simulink library "MSMLib"  (R2018b)
settings: Solver=VariableStepAuto  StartTime=0.0  StopTime=10.0  RelTol=1e-3
undefined symbols (not defined in the file or in its folder): MdTp1, ModeAdjustTp1, PosCallSts1
settings Model: Creator=s69u2m  LastModifiedBy=su3dcu
settings DataIOCC: ReturnWorkspaceOutputs=on

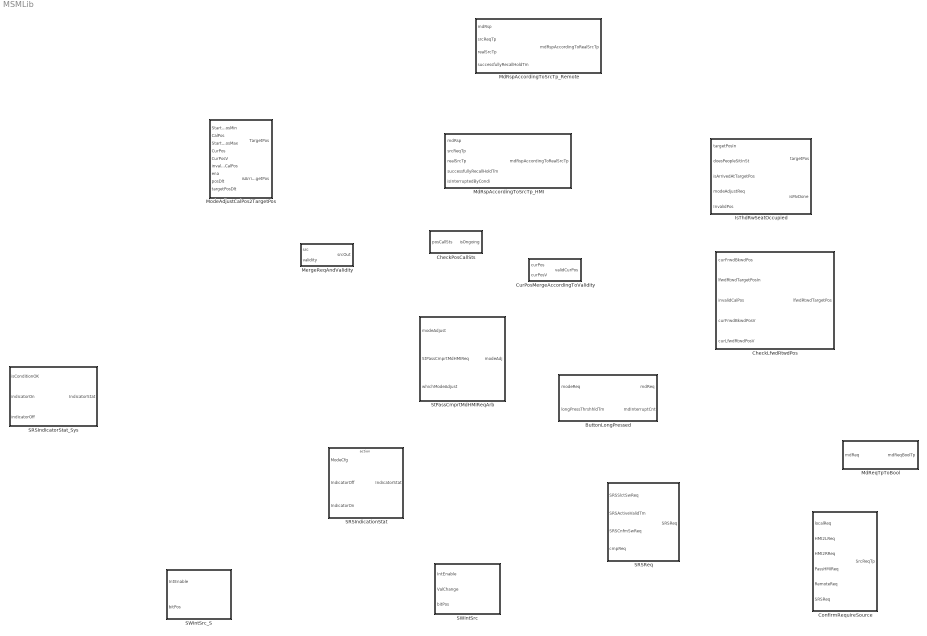
== system MSMLib ==
  ButtonLongPressed : Subsystem
  CheckLfwdRtwdPos : Subsystem
  CheckPosCallSts : Subsystem
  ConfirmRequireSource : Subsystem
  CurPosMergeAccordingToValidity : Subsystem
  IsThdRwSeatOccupied : Subsystem
  MdReqTpToBool : Subsystem
  MdRspAccordingToSrcTp_HMI : Subsystem
  MdRspAccordingToSrcTp_Remote : Subsystem
  MergeReqAndValidity : Subsystem
  ModeAdjustCalPos2TargetPos : Subsystem
  "SRSIndicationStat " : Subsystem  TreatAsAtomicUnit=on
  SRSIndicatorStat_Sys : Subsystem
  SRSReq : Subsystem
  SWIntSrc : Subsystem
  SWIntSrc_S : Subsystem
  StPassCmprtMdHMIReqArb : Subsystem

== system MSMLib/ButtonLongPressed ==
  modeReq : Inport
  longPressThrshhldTm : Inport  Port=2
  Chart1 : Stateflow chart  TreatAsAtomicUnit=on
  mdReq : Outport
  mdInterruptCnt : Outport  Port=2
  wires:
  longPressThrshhldTm/1 -> Chart1/2(iLongPressThrshhldTm)
  Chart1/2(oMdInterruptCnt) -> mdInterruptCnt/1
  Chart1/1(oMdReq) -> mdReq/1
  modeReq/1 -> Chart1/1(iSrc)

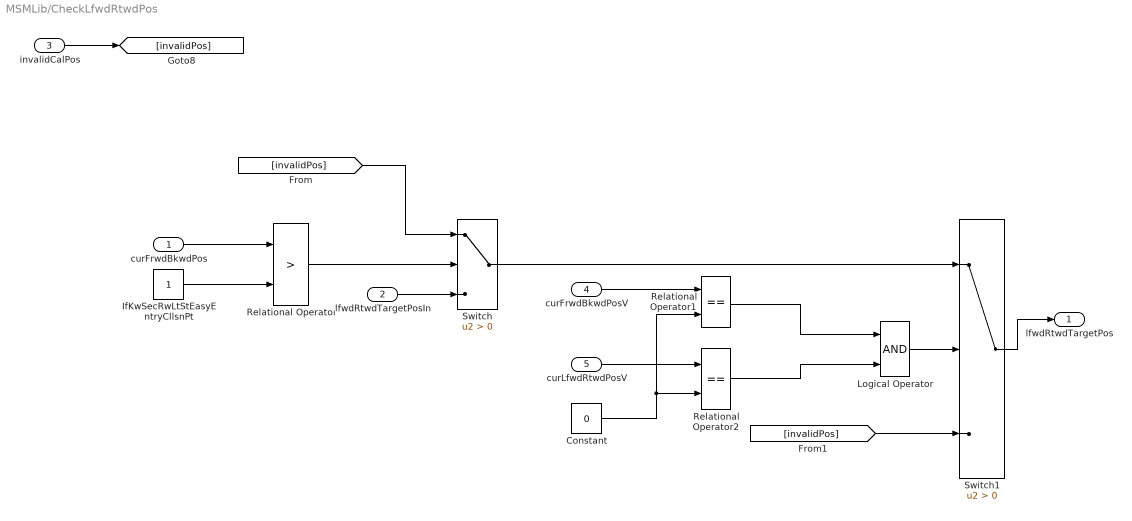
== system MSMLib/CheckLfwdRtwdPos ==
  curFrwdBkwdPos : Inport
  lfwdRtwdTargetPosIn : Inport  Port=2
  invalidCalPos : Inport  Port=3
  curFrwdBkwdPosV : Inport  Port=4
  curLfwdRtwdPosV : Inport  Port=5
  Constant : Constant  Value=0  OutDataTypeStr=uint8
  IfKwSecRwLtStEasyEntryCllsnPt : Constant  OutDataTypeStr=uint16
  Logical Operator : Logic  AllPortsSameDT=off  OutDataTypeStr=boolean
  Relational Operator : RelationalOperator  Operator=>  OutDataTypeStr=boolean  RndMeth=Simplest
  Relational Operator1 : RelationalOperator  Operator===  OutDataTypeStr=boolean  RndMeth=Simplest
  Relational Operator2 : RelationalOperator  Operator===  OutDataTypeStr=boolean  RndMeth=Simplest
  Switch : Switch  Criteria=u2 > Threshold
  Switch1 : Switch  Criteria=u2 > Threshold
  lfwdRtwdTargetPos : Outport  VectorParamsAs1DForOutWhenUnconnected=on
  wires:
  Logical Operator/1 -> Switch1/2
  Relational Operator2/1 -> Logical Operator/2
  curLfwdRtwdPosV/1 -> Relational Operator2/1
  [invalidPos] -> Switch1/3
  Relational Operator1/1 -> Logical Operator/1
  Switch1/1 -> lfwdRtwdTargetPos/1
  Switch/1 -> Switch1/1
  [invalidPos] -> Switch/1
  lfwdRtwdTargetPosIn/1 -> Switch/3
  Relational Operator/1 -> Switch/2
  invalidCalPos/1 -> [invalidPos]
  IfKwSecRwLtStEasyEntryCllsnPt/1 -> Relational Operator/2
  curFrwdBkwdPos/1 -> Relational Operator/1
  curFrwdBkwdPosV/1 -> Relational Operator1/1
  Constant/1 -> Relational Operator1/2, Relational Operator2/2

== system MSMLib/CheckPosCallSts ==
  posCallSts : Inport
  Constant : Constant  Value=PosCallSts1.PosCallSts_Ongoing  OutDataTypeStr=Enum:PosCallSts1
  Relational Operator : RelationalOperator  Operator===  OutDataTypeStr=boolean  RndMeth=Simplest
  isOngoing : Outport  VectorParamsAs1DForOutWhenUnconnected=on
  wires:
  Constant/1 -> Relational Operator/2
  posCallSts/1 -> Relational Operator/1
  Relational Operator/1 -> isOngoing/1

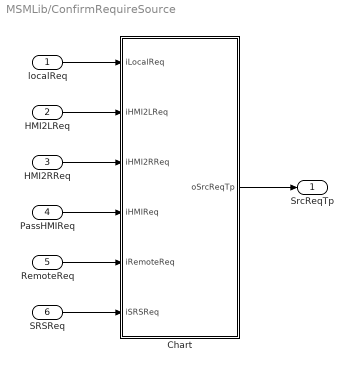
== system MSMLib/ConfirmRequireSource ==
  localReq : Inport
  HMI2LReq : Inport  Port=2
  HMI2RReq : Inport  Port=3
  PassHMIReq : Inport  Port=4
  RemoteReq : Inport  Port=5
  SRSReq : Inport  Port=6
  Chart : Stateflow chart  TreatAsAtomicUnit=on
  SrcReqTp : Outport
  wires:
  HMI2LReq/1 -> Chart/2(iHMI2LReq)
  localReq/1 -> Chart/1(iLocalReq)
  Chart/1(oSrcReqTp) -> SrcReqTp/1
  PassHMIReq/1 -> Chart/4(iHMIReq)
  HMI2RReq/1 -> Chart/3(iHMI2RReq)
  RemoteReq/1 -> Chart/5(iRemoteReq)
  SRSReq/1 -> Chart/6(iSRSReq)

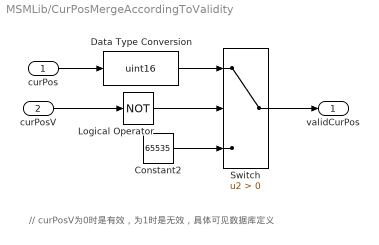
== system MSMLib/CurPosMergeAccordingToValidity ==
  note: // curPosV为0时是有效，为1时是无效，具体可见数据库定义
  curPos : Inport
  curPosV : Inport  Port=2
  Constant2 : Constant  Value=65535  OutDataTypeStr=uint16
  Data Type Conversion : DataTypeConversion  OutDataTypeStr=uint16
  Logical Operator : Logic  Operator=NOT  AllPortsSameDT=off  OutDataTypeStr=boolean
  Switch : Switch  Criteria=u2 > Threshold
  validCurPos : Outport  VectorParamsAs1DForOutWhenUnconnected=on
  wires:
  Constant2/1 -> Switch/3
  Logical Operator/1 -> Switch/2
  Data Type Conversion/1 -> Switch/1
  curPos/1 -> Data Type Conversion/1
  curPosV/1 -> Logical Operator/1
  Switch/1 -> validCurPos/1

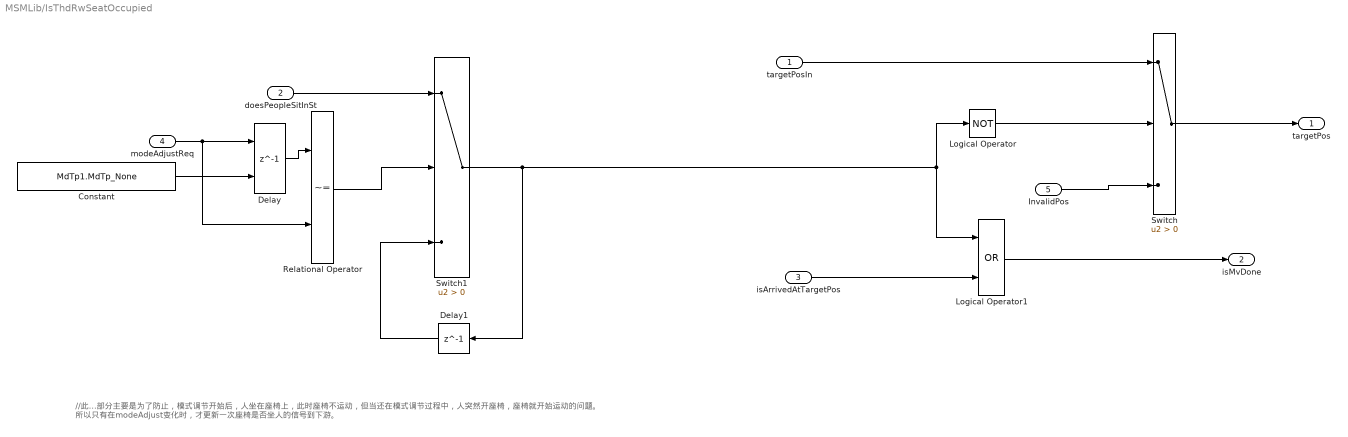
== system MSMLib/IsThdRwSeatOccupied ==
  note: //此部分主要是为了防止，模式调节开始后，人坐在座椅上，此时座椅不运动，但当还在模式调节过程中，人突然开座椅，座椅就开始运动的问题。
      | 所以只有在modeAdjust变化时，才更新一次座椅是否坐人的信号到下游。
  targetPosIn : Inport
  doesPeopleSitInSt : Inport  Port=2
  isArrivedAtTargetPos : Inport  Port=3
  modeAdjustReq : Inport  Port=4
  InvalidPos : Inport  Port=5
  Constant : Constant  Value=MdTp1.MdTp_None  OutDataTypeStr=Enum:MdTp1
  Delay : Delay  DelayLength=1  InitialConditionSource=Input port
      settings: InputPortMap=u0,p4
  Delay1 : Delay  DelayLength=1
  Logical Operator : Logic  Operator=NOT  AllPortsSameDT=off  OutDataTypeStr=boolean
  Logical Operator1 : Logic  Operator=OR  AllPortsSameDT=off  OutDataTypeStr=boolean
  Relational Operator : RelationalOperator  Operator=~=  OutDataTypeStr=boolean  RndMeth=Simplest
  Switch : Switch  Criteria=u2 > Threshold
  Switch1 : Switch  Criteria=u2 > Threshold
  targetPos : Outport  VectorParamsAs1DForOutWhenUnconnected=on
  isMvDone : Outport  Port=2  VectorParamsAs1DForOutWhenUnconnected=on
  wires:
  Switch/1 -> targetPos/1
  Logical Operator1/1 -> isMvDone/1
  isArrivedAtTargetPos/1 -> Logical Operator1/2
  InvalidPos/1 -> Switch/3
  Logical Operator/1 -> Switch/2
  targetPosIn/1 -> Switch/1
  modeAdjustReq/1 -> Relational Operator/2, Delay/1
  Delay/1 -> Relational Operator/1
  Relational Operator/1 -> Switch1/2
  doesPeopleSitInSt/1 -> Switch1/1
  Switch1/1 -> Logical Operator/1, Logical Operator1/1, Delay1/1
  Delay1/1 -> Switch1/3
  Constant/1 -> Delay/2

== system MSMLib/MdReqTpToBool ==
  mdReq : Inport
  Chart : Stateflow chart  TreatAsAtomicUnit=on
  mdReqBoolTp : Outport
  wires:
  Chart/1(oMdReqBool) -> mdReqBoolTp/1
  mdReq/1 -> Chart/1(iMdReq)

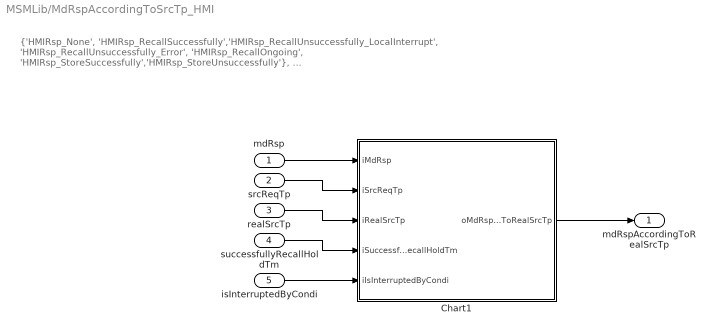
== system MSMLib/MdRspAccordingToSrcTp_HMI ==
  note: {'HMIRsp_None', 'HMIRsp_RecallSuccessfully','HMIRsp_RecallUnsuccessfully_LocalInterrupt', 'HMIRsp_RecallUnsuccessfully_Error', 'HMIRsp_RecallOngoing', 'HMIRsp_StoreSuccessfully','HMIRsp_StoreUnsuccessfully'}, ...
  mdRsp : Inport
  srcReqTp : Inport  Port=2
  realSrcTp : Inport  Port=3
  successfullyRecallHoldTm : Inport  Port=4
  isInterruptedByCondi : Inport  Port=5
  Chart1 : Stateflow chart  TreatAsAtomicUnit=on
  mdRspAccordingToRealSrcTp : Outport
  wires:
  mdRsp/1 -> Chart1/1(iMdRsp)
  srcReqTp/1 -> Chart1/2(iSrcReqTp)
  realSrcTp/1 -> Chart1/3(iRealSrcTp)
  successfullyRecallHoldTm/1 -> Chart1/4(iSuccessfulRecallHoldTm)
  Chart1/1(oMdRspAccordingToRealSrcTp) -> mdRspAccordingToRealSrcTp/1
  isInterruptedByCondi/1 -> Chart1/5(iIsInterruptedByCondi)

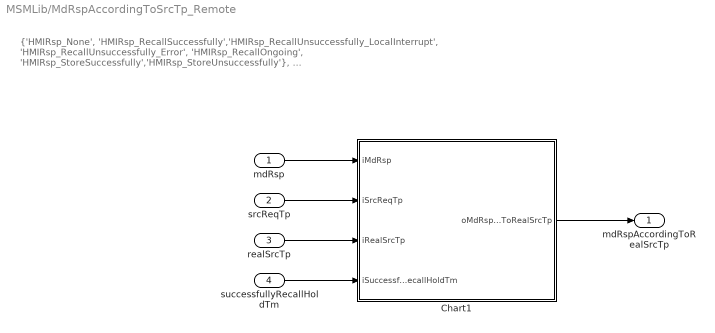
== system MSMLib/MdRspAccordingToSrcTp_Remote ==
  note: {'HMIRsp_None', 'HMIRsp_RecallSuccessfully','HMIRsp_RecallUnsuccessfully_LocalInterrupt', 'HMIRsp_RecallUnsuccessfully_Error', 'HMIRsp_RecallOngoing', 'HMIRsp_StoreSuccessfully','HMIRsp_StoreUnsuccessfully'}, ...
  mdRsp : Inport
  srcReqTp : Inport  Port=2
  realSrcTp : Inport  Port=3
  successfullyRecallHoldTm : Inport  Port=4
  Chart1 : Stateflow chart  TreatAsAtomicUnit=on
  mdRspAccordingToRealSrcTp : Outport
  wires:
  Chart1/1(oMdRspAccordingToRealSrcTp) -> mdRspAccordingToRealSrcTp/1
  successfullyRecallHoldTm/1 -> Chart1/4(iSuccessfulRecallHoldTm)
  realSrcTp/1 -> Chart1/3(iRealSrcTp)
  srcReqTp/1 -> Chart1/2(iSrcReqTp)
  mdRsp/1 -> Chart1/1(iMdRsp)

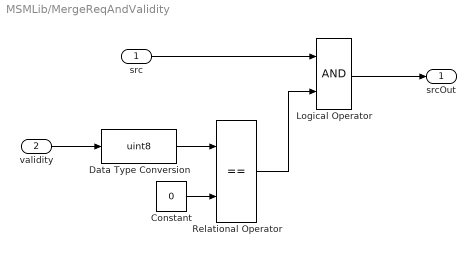
== system MSMLib/MergeReqAndValidity ==
  src : Inport
  validity : Inport  Port=2
  Constant : Constant  Value=0  OutDataTypeStr=uint8
  Data Type Conversion : DataTypeConversion  OutDataTypeStr=uint8
  Logical Operator : Logic  AllPortsSameDT=off  OutDataTypeStr=boolean
  Relational Operator : RelationalOperator  Operator===  OutDataTypeStr=boolean  RndMeth=Simplest
  srcOut : Outport  VectorParamsAs1DForOutWhenUnconnected=on
  wires:
  Relational Operator/1 -> Logical Operator/2
  Logical Operator/1 -> srcOut/1
  validity/1 -> Data Type Conversion/1
  Constant/1 -> Relational Operator/2
  src/1 -> Logical Operator/1
  Data Type Conversion/1 -> Relational Operator/1

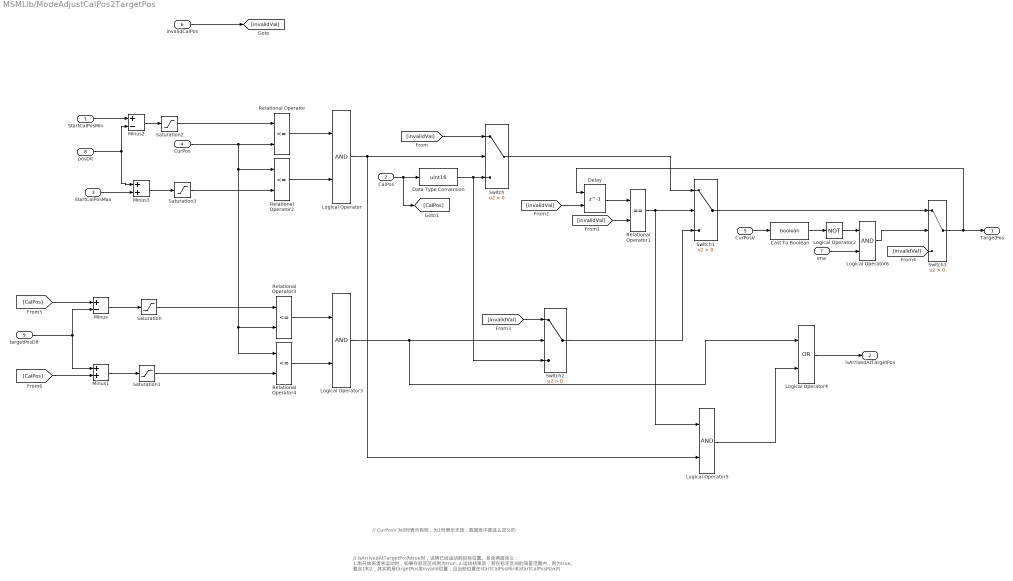
== system MSMLib/ModeAdjustCalPos2TargetPos ==
  note: // isArrivedAtTargetPos为true时，说明已经运动到目标位置。包含两层含义：
      | 1.刚开始来请求运动时，如果在标定区间则为true;
      | 2.运动结束后，若在标定区间的误差范围内，则为true。
      | 整合1和2，其实就是targetPos发invalid位置，且当前位置在startCalPosMin和startCalPosMax内
  note: // CurPosV 为0时表示有效，为1时表示无效，数据库中是这么定义的
  StartCalPosMin : Inport
  CalPos : Inport  Port=2
  StartCalPosMax : Inport  Port=3
  CurPos : Inport  Port=4
  CurPosV : Inport  Port=5
  invalidCalPos : Inport  Port=6
  ena : Inport  Port=7
  posDlt : Inport  Port=8
  targetPosDlt : Inport  Port=9
  Cast To Boolean : DataTypeConversion  OutDataTypeStr=boolean
  Data Type Conversion : DataTypeConversion  OutDataTypeStr=uint16
  Delay : Delay  DelayLength=1  InitialConditionSource=Input port
      settings: InputPortMap=u0,p4
  Logical Operator{,3,5..6} (4 alike) : Logic  AllPortsSameDT=off  OutDataTypeStr=boolean
  Logical Operator2 : Logic  Operator=NOT  AllPortsSameDT=off  OutDataTypeStr=boolean
  Logical Operator4 : Logic  Operator=OR  AllPortsSameDT=off  OutDataTypeStr=boolean
  Minus : Sum  Inputs=+-  OutDataTypeStr=int16
  Minus1 : Sum  OutDataTypeStr=int16
  Minus2 : Sum  Inputs=+-  OutDataTypeStr=int16
  Minus3 : Sum  OutDataTypeStr=uint16
  Relational Operator{,2..4} (4 alike) : RelationalOperator  Operator=<=  OutDataTypeStr=boolean  RndMeth=Simplest
  Relational Operator1 : RelationalOperator  Operator===  OutDataTypeStr=boolean  RndMeth=Simplest
  Saturation : Saturate  UpperLimit=4000  LowerLimit=0  OutDataTypeStr=uint16
  Saturation1 : Saturate  UpperLimit=4000  LowerLimit=0  OutDataTypeStr=uint16
  Saturation2 : Saturate  UpperLimit=4095  LowerLimit=0  OutDataTypeStr=uint16
  Saturation3 : Saturate  UpperLimit=4095  LowerLimit=0  OutDataTypeStr=uint16
  Switch{,1..3} (4 alike) : Switch  Criteria=u2 > Threshold
  TargetPos : Outport  VectorParamsAs1DForOutWhenUnconnected=on
  isArrivedAtTargetPos : Outport  Port=2  VectorParamsAs1DForOutWhenUnconnected=on
  wires:
  StartCalPosMin/1 -> Minus2/1
  Relational Operator/1 -> Logical Operator/1
  StartCalPosMax/1 -> Minus3/2
  Relational Operator2/1 -> Logical Operator/2
  [invalidVal] -> Switch/1
  Logical Operator/1 -> Logical Operator5/2, Switch/2
  Switch/1 -> Switch1/1
  CurPosV/1 -> Cast To Boolean/1
  Cast To Boolean/1 -> Logical Operator2/1
  CalPos/1 -> [CalPos], Data Type Conversion/1
  Delay/1 -> Relational Operator1/1
  Relational Operator1/1 -> Logical Operator5/1, Switch1/2
  Relational Operator3/1 -> Logical Operator3/1
  Relational Operator4/1 -> Logical Operator3/2
  Saturation1/1 -> Relational Operator4/2
  CurPos/1 -> Relational Operator2/1, Relational Operator3/2, Relational Operator4/1, Relational Operator/2
  Saturation/1 -> Relational Operator3/1
  Logical Operator3/1 -> Logical Operator4/1, Switch2/2
  Switch2/1 -> Switch1/3
  Switch1/1 -> Switch3/1
  invalidCalPos/1 -> [invalidVal]
  [invalidVal] -> Relational Operator1/2
  [invalidVal] -> Delay/2
  [invalidVal] -> Switch2/1
  Logical Operator2/1 -> Logical Operator6/1
  [invalidVal] -> Switch3/3
  Data Type Conversion/1 -> Switch/3, Switch2/3
  [CalPos] -> Minus/1
  [CalPos] -> Minus1/2
  Minus/1 -> Saturation/1
  Minus1/1 -> Saturation1/1
  Logical Operator4/1 -> isArrivedAtTargetPos/1
  Logical Operator5/1 -> Logical Operator4/2
  ena/1 -> Logical Operator6/2
  Switch3/1 -> Delay/1, TargetPos/1
  Logical Operator6/1 -> Switch3/2
  targetPosDlt/1 -> Minus1/1, Minus/2
  posDlt/1 -> Minus2/2, Minus3/1
  Minus2/1 -> Saturation2/1
  Saturation2/1 -> Relational Operator/1
  Minus3/1 -> Saturation3/1
  Saturation3/1 -> Relational Operator2/2

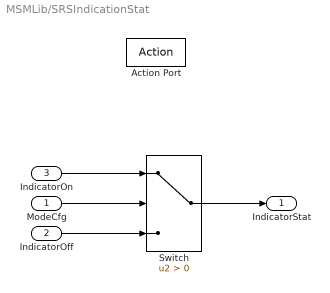
== system MSMLib/SRSIndicationStat  ==
  "ModeCfg " : Inport
  IndicatorOff : Inport  Port=2
  IndicatorOn : Inport  Port=3
  Action Port : ActionPort
  Switch : Switch  Criteria=u2 > Threshold
  "IndicatorStat " : Outport
  wires:
  IndicatorOn/1 -> Switch/1
  "ModeCfg "/1 -> Switch/2
  IndicatorOff/1 -> Switch/3
  Switch/1 -> "IndicatorStat "/1

== system MSMLib/SRSIndicatorStat_Sys ==
  isConditionOK : Inport
  indicatorOn : Inport  Port=2
  indicatorOff : Inport  Port=3
  IndicatorStat_Chart : Stateflow chart  TreatAsAtomicUnit=on
  IndicatorStat : Outport
  wires:
  isConditionOK/1 -> IndicatorStat_Chart/1(isConditionOK)
  indicatorOn/1 -> IndicatorStat_Chart/2(iIndicatorOn)
  indicatorOff/1 -> IndicatorStat_Chart/3(iIndicatorOff)
  IndicatorStat_Chart/1(oIndicatorStat) -> IndicatorStat/1

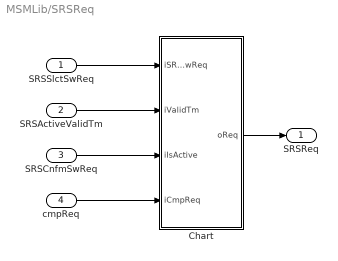
== system MSMLib/SRSReq ==
  SRSSlctSwReq : Inport
  SRSActiveValidTm : Inport  Port=2
  SRSCnfmSwReq : Inport  Port=3
  cmpReq : Inport  Port=4
  Chart : Stateflow chart  TreatAsAtomicUnit=on
  SRSReq : Outport
  wires:
  SRSSlctSwReq/1 -> Chart/1(iSRSSlcSwReq)
  SRSActiveValidTm/1 -> Chart/2(iValidTm)
  SRSCnfmSwReq/1 -> Chart/3(iIsActive)
  cmpReq/1 -> Chart/4(iCmpReq)
  Chart/1(oReq) -> SRSReq/1

== system MSMLib/SWIntSrc ==
  IntEnable : Inport
  "ValChange " : Inport  Port=2
  bitPos : Inport  Port=3
  Chart : Stateflow chart  TreatAsAtomicUnit=on
  wires:
  "ValChange "/1 -> Chart/2(iValChange)
  IntEnable/1 -> Chart/1(iIntEnable)
  bitPos/1 -> Chart/3(ibit)

== system MSMLib/SWIntSrc_S ==
  IntEnable : Inport
  bitPos : Inport  Port=2
  Chart : Stateflow chart  TreatAsAtomicUnit=on
  wires:
  bitPos/1 -> Chart/2(ibit)
  IntEnable/1 -> Chart/1(iIntEnable)

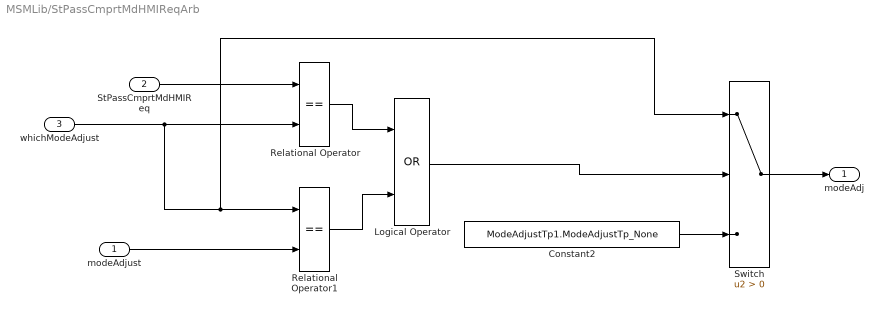
== system MSMLib/StPassCmprtMdHMIReqArb ==
  modeAdjust : Inport
  StPassCmprtMdHMIReq : Inport  Port=2
  whichModeAdjust : Inport  Port=3
  Constant2 : Constant  Value=ModeAdjustTp1.ModeAdjustTp_None  OutDataTypeStr=Enum:ModeAdjustTp1
  Logical Operator : Logic  Operator=OR  AllPortsSameDT=off  OutDataTypeStr=boolean
  Relational Operator : RelationalOperator  Operator===  OutDataTypeStr=boolean  RndMeth=Simplest
  Relational Operator1 : RelationalOperator  Operator===  OutDataTypeStr=boolean  RndMeth=Simplest
  Switch : Switch  Criteria=u2 > Threshold
  modeAdj : Outport  VectorParamsAs1DForOutWhenUnconnected=on
  wires:
  Relational Operator/1 -> Logical Operator/1
  StPassCmprtMdHMIReq/1 -> Relational Operator/1
  Switch/1 -> modeAdj/1
  whichModeAdjust/1 -> Switch/1, Relational Operator1/1, Relational Operator/2
  modeAdjust/1 -> Relational Operator1/2
  Relational Operator1/1 -> Logical Operator/2
  Logical Operator/1 -> Switch/2
  Constant2/1 -> Switch/3

== system MSMLib/SWIntSrc/Chart/MdSWIntSrc_Get ==
  f : TriggerPort  TriggerType=function-call  VariantControl=(inherit)
      settings: CopyFcn=Stateflow.SLINSF.SimulinkMan.removeBlockPreDeleteFcn  PreDeleteFcn=Stateflow.SLINSF.SimulinkMan.unsafePredeleteFcn
  Data Store Read : DataStoreRead  DataStoreName=MdSWIntSrc_Val
  data : Outport  OutDataTypeStr=uint16  PortDimensions=1  SampleTime=0.01
  wires:
  Data Store Read/1 -> data/1

== system MSMLib/SWIntSrc/Chart/MdSWIntSrc_Set ==
  data : Inport  OutDataTypeStr=uint16  PortDimensions=1  SampleTime=0.01
  f : TriggerPort  TriggerType=function-call  VariantControl=(inherit)
      settings: CopyFcn=Stateflow.SLINSF.SimulinkMan.removeBlockPreDeleteFcn  PreDeleteFcn=Stateflow.SLINSF.SimulinkMan.unsafePredeleteFcn
  Data Store Write : DataStoreWrite  DataStoreName=MdSWIntSrc_Val
  wires:
  data/1 -> Data Store Write/1

== system MSMLib/SWIntSrc_S/Chart/MdSWIntSrc_Get ==
  f : TriggerPort  TriggerType=function-call  VariantControl=(inherit)
      settings: CopyFcn=Stateflow.SLINSF.SimulinkMan.removeBlockPreDeleteFcn  PreDeleteFcn=Stateflow.SLINSF.SimulinkMan.unsafePredeleteFcn
  Data Store Read : DataStoreRead  DataStoreName=MdSWIntSrc_Val
  data : Outport  OutDataTypeStr=uint16  PortDimensions=1  SampleTime=0.01
  wires:
  Data Store Read/1 -> data/1

== system MSMLib/SWIntSrc_S/Chart/MdSWIntSrc_Set ==
  data : Inport  OutDataTypeStr=uint16  PortDimensions=1  SampleTime=0.01
  f : TriggerPort  TriggerType=function-call  VariantControl=(inherit)
      settings: CopyFcn=Stateflow.SLINSF.SimulinkMan.removeBlockPreDeleteFcn  PreDeleteFcn=Stateflow.SLINSF.SimulinkMan.unsafePredeleteFcn
  Data Store Write : DataStoreWrite  DataStoreName=MdSWIntSrc_Val
  wires:
  data/1 -> Data Store Write/1

== stateflow chart MSMLib/MdRspAccordingToSrcTp_HMI/Chart1 ==
  state RealSrcTp
    state None
      en:
      oMdRspAccordingToRealSrcTp = HMIRsp1.HMIRsp_None;
    state Ongoing
      en:
      oMdRspAccordingToRealSrcTp = HMIRsp1.HMIRsp_RecallOngoing;
    state successful
      en:
      oMdRspAccordingToRealSrcTp = HMIRsp1.HMIRsp_RecallSuccessfully;
    state Unsuccessful
      state Unsuccess
      (default) -> (junction 41)
      (junction 41) -> Unsuccess [order 1] : [iIsInterruptedByCondi]
          | {oMdRspAccordingToRealSrcTp = HMIRsp1.HMIRsp_RecallUnsuccessfully_Error;}
      (junction 41) -> (junction 43) [order 2]
      (junction 43) -> Unsuccess : {oMdRspAccordingToRealSrcTp = HMIRsp1.HMIRsp_RecallUnsuccessfully_LocalInterrupt;}
    (default) -> (junction 20)
    (junction 20) -> None [order 2]
    (junction 20) -> Ongoing [order 1] : [iMdRsp == MdRsp1.MdRsp_RecallOngoing]
    None -> Ongoing : [iMdRsp == MdRsp1.MdRsp_RecallOngoing]
    Ongoing -> Unsuccessful [order 1] : [iMdRsp == MdRsp1.MdRsp_RecallUnsuccessfully]
    Ongoing -> successful [order 2] : [iMdRsp == MdRsp1.MdRsp_RecallSuccessfully]
    Ongoing -> Unsuccess [order 3] : [iSrcReqTp!=iRealSrcTp]
        | {oMdRspAccordingToRealSrcTp = HMIRsp1.HMIRsp_RecallUnsuccessfully_LocalInterrupt}
    successful -> (junction 35) : [after(iSuccessfulRecallHoldTm,tick)]
    Unsuccessful -> (junction 35) : [after(iSuccessfulRecallHoldTm,tick)]
  state Idle
    en:
    oMdRspAccordingToRealSrcTp = MdRsp1.MdRsp_None;
  (default) -> Idle
  Idle -> RealSrcTp : [iSrcReqTp== iRealSrcTp]
  (junction 35) -> Idle
  data: iMdRsp input Enum: MdRsp1; iSrcReqTp input Enum: SrcReqTp1; oMdRspAccordingToRealSrcTp output Enum: HMIRsp1; iRealSrcTp input Enum: SrcReqTp1; iSuccessfulRecallHoldTm input uint8; iIsInterruptedByCondi input boolean

== stateflow chart MSMLib/ButtonLongPressed/Chart1 ==
  state NotPressed
    en:
    oMdReq = false;
  state ButtonPressed
    state idle
    state idle1
      en:
      oMdReq=true;
    (default) -> idle
    idle -> idle1 [order 2] : [after(iLongPressThrshhldTm,tick)]
  (default) -> NotPressed : {oMdInterruptCnt = 0;}
  NotPressed -> ButtonPressed : [hasChangedTo(iSrc, true)]
  idle -> NotPressed [order 1] : [!iSrc]
      | {oMdInterruptCnt ++;}
  idle1 -> NotPressed : [!iSrc]
  data: iSrc input boolean; oMdReq output boolean; oMdInterruptCnt output uint8; iLongPressThrshhldTm input uint8

== stateflow chart MSMLib/MdReqTpToBool/Chart ==
  state Idle
  state Stop
  state Start
    en:
    oMdReqBool = true;
    ex:
    oMdReqBool = false;
  state Cancel
  (default) -> Idle
  Idle -> Start : [iMdReq ==  MdReqTp1.MdReqTp_Start]
  Start -> Idle [order 2] : [iMdReq ==  MdReqTp1.MdReqTp_NoAction]
  Stop -> Idle [order 2] : [iMdReq ==  MdReqTp1.MdReqTp_NoAction]
  Cancel -> Idle [order 1] : [iMdReq ==  MdReqTp1.MdReqTp_NoAction]
  Start -> Stop [order 1] : [iMdReq ==  MdReqTp1.MdReqTp_Stop]
  Stop -> Start [order 1] : [iMdReq ==  MdReqTp1.MdReqTp_Start]
  Start -> Cancel [order 3] : [iMdReq ==  MdReqTp1.MdReqTp_Cancel]
  Cancel -> Start [order 2] : [iMdReq ==  MdReqTp1.MdReqTp_Start]
  Stop -> Cancel [order 3] : [iMdReq ==  MdReqTp1.MdReqTp_Cancel]
  data: iMdReq input Enum: MdReqTp1; oMdReqBool output boolean

== stateflow chart MSMLib/SRSReq/Chart ==
  state SRSNonAvail
    en:
    oReq = false;
  state SRSAvail
    state NonActive
      en:
      oReq = false;
    state Active
      en:
      oReq = true;
    (default) -> NonActive
    NonActive -> SRSAvail.Active [order 1] : [hasChangedTo(iIsActive,true)]
  state None [commented out]
    en:
    oReq = false;
  state SelectedMd [commented out]
    state dle [commented out]
      en:
      oReq=false;
    state Active [commented out]
      en:
      oReq = true;
    (default) -> dle [commented out]
    dle -> SelectedMd.Active [commented out] : [iIsActive]
    SelectedMd.Active -> dle [commented out] : [!iIsActive]
  (default) -> SRSNonAvail
  SRSNonAvail -> NonActive : [hasChangedTo(iSRSSlcSwReq,iCmpReq)]
  NonActive -> SRSNonAvail [order 2] : [after(iValidTm,tick) || ...
      | ((iSRSSlcSwReq != iCmpReq) && (iSRSSlcSwReq != SRSMode1.SRSSlctSwStat_None))]
  SRSAvail.Active -> SRSNonAvail : [after(3,tick)]
  (default) -> None [commented out]
  None -> SelectedMd [commented out] : [hasChangedTo(iSRSSlcSwReq, iCmpReq)]
  dle -> None [commented out] : [after(iValidTm,tick)]
  SelectedMd -> None [commented out] : [iSRSSlcSwReq != iCmpReq]
  data: iSRSSlcSwReq input Enum: SRSMode1; iValidTm input uint16; iIsActive input boolean; iCmpReq input Enum: SRSMode1; oReq output boolean

== stateflow chart MSMLib/MdRspAccordingToSrcTp_Remote/Chart1 ==
  state RealSrcTp
    state None
      en:
      oMdRspAccordingToRealSrcTp = PassRsp1.PassRsp_None;
    state Ongoing
      en:
      oMdRspAccordingToRealSrcTp = PassRsp1.PassRsp_Ongoing;
    state successful
      en:
      oMdRspAccordingToRealSrcTp = PassRsp1.PassRsp_RecallSuccessfully;
    state Unsuccessful
      en:
      oMdRspAccordingToRealSrcTp = PassRsp1.PassRsp_RecallUnSuccessfully;
    (default) -> (junction 20)
    (junction 20) -> None [order 2]
    (junction 20) -> Ongoing [order 1] : [iMdRsp == MdRsp1.MdRsp_RecallOngoing]
    None -> Ongoing : [iMdRsp == MdRsp1.MdRsp_RecallOngoing]
    Ongoing -> Unsuccessful [order 1] : [iMdRsp == MdRsp1.MdRsp_RecallUnsuccessfully]
    Ongoing -> Unsuccessful [order 3] : [iSrcReqTp!=iRealSrcTp]
    Ongoing -> successful [order 2] : [iMdRsp == MdRsp1.MdRsp_RecallSuccessfully]
    successful -> (junction 35) : [after(iSuccessfulRecallHoldTm,tick)]
    Unsuccessful -> (junction 35) : [after(iSuccessfulRecallHoldTm,tick)]
  state Idle
    en:
    oMdRspAccordingToRealSrcTp = MdRsp1.MdRsp_None;
  (default) -> Idle
  Idle -> RealSrcTp : [iSrcReqTp==iRealSrcTp]
  (junction 35) -> Idle
  data: iMdRsp input Enum: MdRsp1; iSrcReqTp input Enum: SrcReqTp1; oMdRspAccordingToRealSrcTp output Enum: PassRsp1; iRealSrcTp input Enum: SrcReqTp1; iSuccessfulRecallHoldTm input uint8

== stateflow chart MSMLib/SWIntSrc_S/Chart ==
  state data = MdSWIntSrc_Get [function]
  state MdSWIntSrc_Set(data) [function]
  (default) -> (junction 41)
  (junction 41) -> (junction 43) [order 1] : [iIntEnable == true]
  (junction 41) -> (junction 48) [order 2]
  (junction 43) -> (junction 46) : {SWIntSrc = MdSWIntSrc_Get();
      | SWIntSrc |= (0x1<<(ibit&0xf));
      | i_flag = true;}
  (junction 48) -> (junction 51) [order 1] : [i_flag == true]
  (junction 48) -> (junction 52) [order 2]
  (junction 51) -> (junction 55) : {SWIntSrc = MdSWIntSrc_Get();
      | SWIntSrc &= (~(0x1<<(ibit&0xf)));
      | i_flag = false;}
  (junction 55) -> (junction 52) : {MdSWIntSrc_Set(SWIntSrc);}
  (junction 46) -> (junction 55)
  (junction 52) -> (junction 59)
  data: data function_output uint16 size=1; data function_input uint16 size=1; iIntEnable input boolean size=1; SWIntSrc local uint16 size=1; ibit input uint8; i_flag local boolean size=1

== stateflow chart MSMLib/SRSIndicatorStat_Sys/IndicatorStat_Chart ==
  state Off
    en:
    oIndicatorStat = iIndicatorOff;
  state On
    en:
    oIndicatorStat = iIndicatorOn;
  (default) -> Off
  Off -> On : [hasChangedTo(isConditionOK, true)]
  On -> Off : [!isConditionOK]
  data: isConditionOK input boolean; iIndicatorOn input Enum: SRSIndicatorStat1; iIndicatorOff input Enum: SRSIndicatorStat1; oIndicatorStat output Enum: SRSIndicatorStat1

== stateflow chart MSMLib/ConfirmRequireSource/Chart ==
  state None [commented out]
    en:
    oSrcReqTp = SrcReqTp1.SrcReqTp_None;
  state SRS [commented out]
    en:
    oSrcReqTp = SrcReqTp1.SrcReqTp_SRS;
  state Local [commented out]
    en:
    oSrcReqTp = SrcReqTp1.SrcReqTp_Local;
  state Remote [commented out]
    en:
    oSrcReqTp = SrcReqTp1.SrcReqTp_Remote;
  state HMI2L [commented out]
    en:
    oSrcReqTp = SrcReqTp1.SrcReqTp_HMI2L;
  state HMI [commented out]
    en:
    oSrcReqTp = SrcReqTp1.SrcReqTp_HMI;
  state HMI2R [commented out]
    en:
    oSrcReqTp = SrcReqTp1.SrcReqTp_HMI2R;
  state out = FindReqSrc [function]
    note: [iLocalReq||...
        | iHMI2LReq||...
        | iHMI2RReq||...
        | iHMIReq||...
        | iRemoteReq]
    (default) -> (junction 194)
    (junction 194) -> (junction 196) [order 1] : [hasChangedTo(iLocalReq,true)]
    (junction 194) -> (junction 200) [order 2]
    (junction 196) -> (junction 198) : {out = SrcReqTp1.SrcReqTp_Local;}
    (junction 200) -> (junction 202) [order 1] : [hasChangedTo(iHMI2LReq,true)]
    (junction 200) -> (junction 206) [order 2]
    (junction 202) -> (junction 204) : {out = SrcReqTp1.SrcReqTp_HMI2L;}
    (junction 206) -> (junction 208) [order 1] : [hasChangedTo(iHMI2RReq, true)]
    (junction 206) -> (junction 251) [order 2]
    (junction 208) -> (junction 210) : {out = SrcReqTp1.SrcReqTp_HMI2R;}
    (junction 251) -> (junction 252) [order 1] : [hasChangedTo(iSRSReq, true)]
    (junction 251) -> (junction 218) [order 2]
    (junction 252) -> (junction 256) : {out = SrcReqTp1.SrcReqTp_SRS;}
    (junction 218) -> (junction 220) [order 1] : [hasChangedTo(iHMIReq, true)]
    (junction 218) -> (junction 224) [order 2]
    (junction 220) -> (junction 222) : {out = SrcReqTp1.SrcReqTp_HMI;}
    (junction 224) -> (junction 226) [order 1] : [hasChangedTo(iRemoteReq, true)]
    (junction 224) -> (junction 228) [order 2] : {out = SrcReqTp1.SrcReqTp_None;}
    (junction 226) -> (junction 231) : {out = SrcReqTp1.SrcReqTp_Remote;}
    (junction 231) -> (junction 228)
    (junction 222) -> (junction 231)
    (junction 256) -> (junction 222)
    (junction 210) -> (junction 256)
    (junction 204) -> (junction 210)
    (junction 198) -> (junction 204)
    (junction 228) -> (junction 239)
  state NoReq
    en:
    oSrcReqTp = SrcReqTp1.SrcReqTp_None;
  state Req
    en:
    oSrcReqTp = FindReqSrc();
  (default) -> None [commented out]
  None -> (junction 1) [commented out] : [iLocalReq||...
      | iHMI2LReq||...
      | iHMI2RReq||...
      | iHMIReq||...
      | iRemoteReq||...
      | iSRSReq]
  (junction 1) -> None [commented out] : [!iLocalReq&&...
      | !iHMI2LReq&&...
      | !iHMI2RReq&&...
      | !iHMIReq&&...
      | !iRemoteReq&&...
      | !iSRSReq]
  (junction 1) -> SRS [commented out] : [iSRSReq]
  SRS -> (junction 1) [commented out] : [intSRS()]
  Remote -> (junction 1) [commented out] : [intRemote()]
  (junction 1) -> Remote [commented out] : [iRemoteReq]
  Local -> (junction 1) [commented out] : [intLocal()]
  (junction 1) -> Local [commented out] : [iLocalReq]
  (junction 1) -> HMI [commented out] : [iHMIReq]
  (junction 1) -> HMI2L [commented out] : [iHMI2LReq]
  HMI2R -> (junction 1) [commented out] : [intHMI2R()]
  HMI -> (junction 1) [commented out] : [intHMI()]
  (junction 1) -> HMI2R [commented out] : [iHMI2RReq]
  HMI2L -> (junction 1) [commented out] : [intHMI2L()]
  (default) -> NoReq
  NoReq -> Req : [iLocalReq||...
      | iHMI2LReq||...
      | iHMI2RReq||...
      | iHMIReq||...
      | iRemoteReq||...
      | iSRSReq]
  Req -> NoReq : [!iLocalReq&&...
      | !iHMI2LReq&&...
      | !iHMI2RReq&&...
      | !iHMIReq&&...
      | !iRemoteReq&&...
      | !iSRSReq]
  data: out function_output Enum: SrcReqTp1; iLocalReq input boolean; iHMI2LReq input boolean; iHMI2RReq input boolean; iHMIReq input boolean; iRemoteReq input boolean; oSrcReqTp output Enum: SrcReqTp1; iSRSReq input boolean

== stateflow chart MSMLib/SWIntSrc/Chart ==
  state data = MdSWIntSrc_Get [function]
  state MdSWIntSrc_Set(data) [function]
  (default) -> (junction 22)
  (junction 22) -> (junction 25) [order 1] : [iValChange == true]
  (junction 22) -> (junction 17) [order 2]
  (junction 25) -> (junction 27) : {SWIntSrc = MdSWIntSrc_Get();}
  (junction 27) -> (junction 29) [order 1] : [iIntEnable == true]
  (junction 27) -> (junction 33) [order 2] : {SWIntSrc &= (~(0x1<<(ibit&0xf)));}
  (junction 29) -> (junction 31) : {SWIntSrc |=(0x1<< (ibit&0xf));}
  (junction 33) -> (junction 17) : {MdSWIntSrc_Set(SWIntSrc);}
  (junction 31) -> (junction 33)
  (junction 17) -> (junction 38)
  data: data function_output uint16 size=1; data function_input uint16 size=1; iIntEnable input boolean; SWIntSrc local uint16 size=1; iValChange input boolean; ibit input uint8
